simulink model "dinpend1"  (R2015a)
settings: Solver=ode45  StartTime=0.0  StopTime=80.0  RelTol=1e-6
settings Model: Creator=jomle  LastModifiedBy=jomle

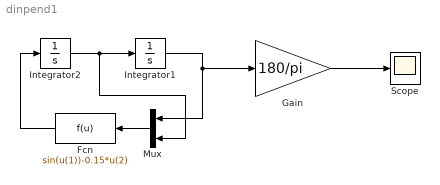
== system dinpend1 ==
  Fcn : Fcn  Expr=sin(u(1))-0.15*u(2)
  Gain : Gain  Gain=180/pi
  Integrator1 : Integrator  InitialCondition=0.001
  Integrator2 : Integrator
  Mux : Mux  Inputs=2
  Scope : Scope
  wires:
  Integrator2/1 -> Mux/2, Integrator1/1
  Integrator1/1 -> Mux/1, Gain/1
  Fcn/1 -> Integrator2/1
  Mux/1 -> Fcn/1
  Gain/1 -> Scope/1
